simulink model "cart_p_step_sim"  (R2013a)
settings: Solver=ode4  StartTime=0.0  StopTime=t_end  FixedStep=0.001  RelTol=1e-3
values from neighbouring files (symbols this model uses):
  ac = 6.25    [p1c62_ex1_cart_p_step.m]    (also in p1c62_ex2_cart_pi_ramp.m; p1c62_ex3_cart_p_step_dis.m; p1c62_ex4_cart_pi_step_dis.m)
  bc = 4.36    [p1c62_ex1_cart_p_step.m]    (also in p1c62_ex2_cart_pi_ramp.m; p1c62_ex3_cart_p_step_dis.m; p1c62_ex4_cart_pi_step_dis.m)
  kP = 10    [p1c62_ex1_cart_p_step.m]    (also in p1c62_ex2_cart_pi_ramp.m; p1c62_ex3_cart_p_step_dis.m; p1c62_ex4_cart_pi_step_dis.m)
  r0 = 0.5    [p1c62_ex1_cart_p_step.m]    (also in p1c62_ex2_cart_pi_ramp.m = 0.1; p1c62_ex3_cart_p_step_dis.m; p1c62_ex4_cart_pi_step_dis.m; p1c63_ex5_cdip_lqr_servo.m)
settings Model: Creator=kawata  LastModifiedBy=kawata

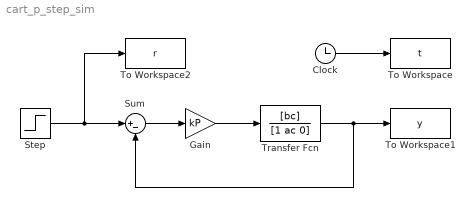
== system cart_p_step_sim ==
  Clock : Clock
  Gain : Gain  Gain=kP
  Step : Step  Time=0  After=r0  SampleTime=0
  Sum : Sum  Inputs=|+-
  To Workspace : ToWorkspace  VariableName=t  SampleTime=-1
  To Workspace1 : ToWorkspace  VariableName=y  SampleTime=-1
  To Workspace2 : ToWorkspace  VariableName=r  SampleTime=-1
  Transfer Fcn : TransferFcn  Numerator=[bc]  Denominator=[1 ac 0]
  wires:
  Step/1 -> To Workspace2/1, Sum/1
  Sum/1 -> Gain/1
  Gain/1 -> Transfer Fcn/1
  Transfer Fcn/1 -> Sum/2, To Workspace1/1
  Clock/1 -> To Workspace/1
